simulink model "vendingMachine"  (R2020b)
settings: Solver=VariableStepAuto  StartTime=0.0  StopTime=200  RelTol=1e-3
settings Model: Creator=baner  LastModifiedBy=baner

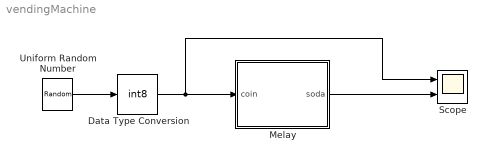
== system vendingMachine ==
  Data Type Conversion : DataTypeConversion  OutDataTypeStr=int8
  "Melay " : Stateflow chart  TreatAsAtomicUnit=on
  Scope : Scope  NumInputPorts=2
  Uniform Random Number : UniformRandomNumber  Minimum=0  Maximum=2  Seed=447  SampleTime=10
  wires:
  Uniform Random Number/1 -> Data Type Conversion/1
  "Melay "/1(soda) -> Scope/2
  Data Type Conversion/1 -> Scope/1, "Melay "/1(coin)

== stateflow chart vendingMachine/Melay  ==
  settings: stateMachineType=MEALY_MACHINE  initializeOutput=1
  note: Soda release on 15 INR
  state got_0
  state got_5_INR
  state got_10_INR
  (default) -> got_0
  got_0 -> got_5_INR [order 1] : [coin==1]{soda=0}
  got_5_INR -> got_0 [order 2] : [coin==2]{soda=1}
  got_5_INR -> got_10_INR [order 1] : [coin==1]{soda=0}
  got_10_INR -> got_5_INR [order 2] : [coin==2]{soda=1}
  got_10_INR -> got_0 [order 1] : [coin==1]{soda=1}
  got_0 -> got_10_INR [order 2] : [coin==2]{soda=0}
  data: coin input int8; soda output boolean
